simulink model "simulation"  (R2018a)
settings: Solver=VariableStepAuto  StartTime=0.0  StopTime=10.0  RelTol=1e-3
libraries: simulink x6
settings Model: Creator=Migue  LastModifiedBy=Migue
settings SolverCC: AlgebraicLoopSolver=LineSearch

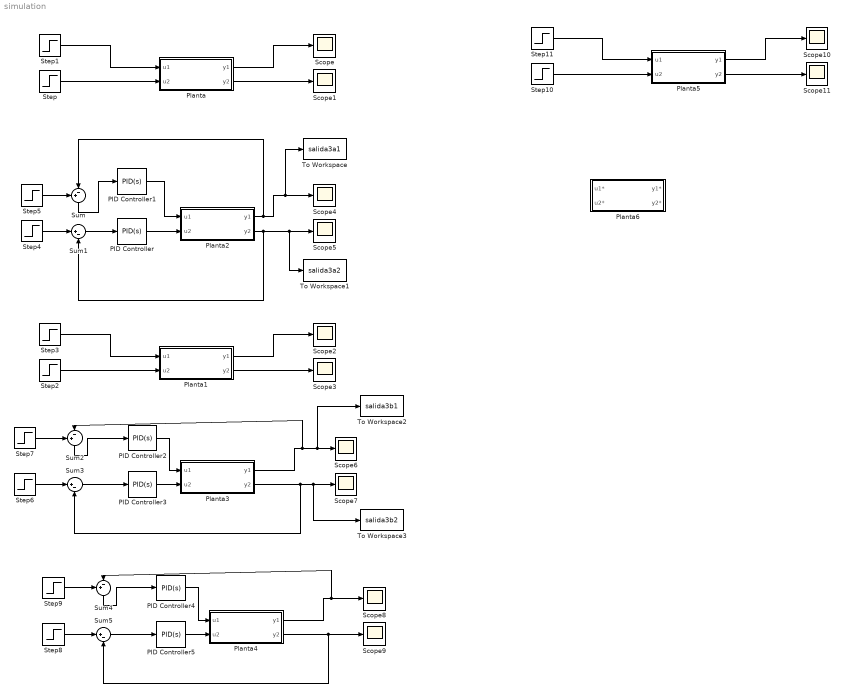
== system simulation ==
  PID Controller : simulink/Continuous/PID Controller  Controller=PID  TimeDomain=Continuous-time  SampleTime=-1  IntegratorMethod=Forward Euler  FilterMethod=Forward Euler  Form=Parallel  UseFilter=on  ControllerParametersSource=internal  P=0  I=19.5  D=0  N=100  InitialConditionSource=internal  InitialConditionForIntegrator=0  InitialConditionForFilter=0  ExternalReset=none  LimitOutput=off  UpperSaturationLimit=inf  LowerSaturationLimit=-inf  LinearizeAsGain=on  AntiWindupMode=none  Kb=1  TrackingMode=off  Kt=1  PParamMin=[]  PParamMax=[]  IParamMin=[]  IParamMax=[]  DParamMin=[]  DParamMax=[]  NParamMin=[]  NParamMax=[]  KbParamMin=[]  KbParamMax=[]  KtParamMin=[]  KtParamMax=[]  POutMin=[]  POutMax=[]  IOutMin=[]  IOutMax=[]  DOutMin=[]  DOutMax=[]  NOutMin=[]  NOutMax=[]  KbOutMin=[]  KbOutMax=[]  KtOutMin=[]  KtOutMax=[]  IntegratorOutMin=[]  IntegratorOutMax=[]  FilterOutMin=[]  FilterOutMax=[]  SumOutMin=[]  SumOutMax=[]  SumI1OutMin=[]  SumI1OutMax=[]  SumI2OutMin=[]  SumI2OutMax=[]  SumI3OutMin=[]  SumI3OutMax=[]  SumDOutMin=[]  SumDOutMax=[]  SaturationOutMin=[]  SaturationOutMax=[]  IntegratorContinuousStateAttributes=''  IntegratorStateMustResolveToSignalObject=off  IntegratorRTWStateStorageClass=Auto  FilterContinuousStateAttributes=''  FilterStateMustResolveToSignalObject=off  FilterRTWStateStorageClass=Auto  DifferentiatorICPrevScaledInput=0  DifferentiatorOutMin=[]  DifferentiatorOutMax=[]  FilterDiffOutCoefMin=[]  FilterDiffOutCoefMax=[]  SumDenOutMin=[]  SumDenOutMax=[]  SumNumOutMin=[]  SumNumOutMax=[]  ReciprocalOutMin=[]  ReciprocalOutMax=[]  DivideOutMin=[]  DivideOutMax=[]  TunerSelectOption=Transfer Function Based (PID Tuner App)
  PID Controller1 : simulink/Continuous/PID Controller  Controller=PID  TimeDomain=Continuous-time  SampleTime=-1  IntegratorMethod=Forward Euler  FilterMethod=Forward Euler  Form=Parallel  UseFilter=on  ControllerParametersSource=internal  P=0  I=9.5  D=0  N=100  InitialConditionSource=internal  InitialConditionForIntegrator=0  InitialConditionForFilter=0  ExternalReset=none  LimitOutput=off  UpperSaturationLimit=inf  LowerSaturationLimit=-inf  LinearizeAsGain=on  AntiWindupMode=none  Kb=1  TrackingMode=off  Kt=1  PParamMin=[]  PParamMax=[]  IParamMin=[]  IParamMax=[]  DParamMin=[]  DParamMax=[]  NParamMin=[]  NParamMax=[]  KbParamMin=[]  KbParamMax=[]  KtParamMin=[]  KtParamMax=[]  POutMin=[]  POutMax=[]  IOutMin=[]  IOutMax=[]  DOutMin=[]  DOutMax=[]  NOutMin=[]  NOutMax=[]  KbOutMin=[]  KbOutMax=[]  KtOutMin=[]  KtOutMax=[]  IntegratorOutMin=[]  IntegratorOutMax=[]  FilterOutMin=[]  FilterOutMax=[]  SumOutMin=[]  SumOutMax=[]  SumI1OutMin=[]  SumI1OutMax=[]  SumI2OutMin=[]  SumI2OutMax=[]  SumI3OutMin=[]  SumI3OutMax=[]  SumDOutMin=[]  SumDOutMax=[]  SaturationOutMin=[]  SaturationOutMax=[]  IntegratorContinuousStateAttributes=''  IntegratorStateMustResolveToSignalObject=off  IntegratorRTWStateStorageClass=Auto  FilterContinuousStateAttributes=''  FilterStateMustResolveToSignalObject=off  FilterRTWStateStorageClass=Auto  DifferentiatorICPrevScaledInput=0  DifferentiatorOutMin=[]  DifferentiatorOutMax=[]  FilterDiffOutCoefMin=[]  FilterDiffOutCoefMax=[]  SumDenOutMin=[]  SumDenOutMax=[]  SumNumOutMin=[]  SumNumOutMax=[]  ReciprocalOutMin=[]  ReciprocalOutMax=[]  DivideOutMin=[]  DivideOutMax=[]  TunerSelectOption=Transfer Function Based (PID Tuner App)
  PID Controller2 : simulink/Continuous/PID Controller  Controller=PID  TimeDomain=Continuous-time  SampleTime=-1  IntegratorMethod=Forward Euler  FilterMethod=Forward Euler  Form=Parallel  UseFilter=on  ControllerParametersSource=internal  P=0.06  I=16.15  D=0  N=100  InitialConditionSource=internal  InitialConditionForIntegrator=0  InitialConditionForFilter=0  ExternalReset=none  LimitOutput=off  UpperSaturationLimit=inf  LowerSaturationLimit=-inf  LinearizeAsGain=on  AntiWindupMode=none  Kb=1  TrackingMode=off  Kt=1  PParamMin=[]  PParamMax=[]  IParamMin=[]  IParamMax=[]  DParamMin=[]  DParamMax=[]  NParamMin=[]  NParamMax=[]  KbParamMin=[]  KbParamMax=[]  KtParamMin=[]  KtParamMax=[]  POutMin=[]  POutMax=[]  IOutMin=[]  IOutMax=[]  DOutMin=[]  DOutMax=[]  NOutMin=[]  NOutMax=[]  KbOutMin=[]  KbOutMax=[]  KtOutMin=[]  KtOutMax=[]  IntegratorOutMin=[]  IntegratorOutMax=[]  FilterOutMin=[]  FilterOutMax=[]  SumOutMin=[]  SumOutMax=[]  SumI1OutMin=[]  SumI1OutMax=[]  SumI2OutMin=[]  SumI2OutMax=[]  SumI3OutMin=[]  SumI3OutMax=[]  SumDOutMin=[]  SumDOutMax=[]  SaturationOutMin=[]  SaturationOutMax=[]  IntegratorContinuousStateAttributes=''  IntegratorStateMustResolveToSignalObject=off  IntegratorRTWStateStorageClass=Auto  FilterContinuousStateAttributes=''  FilterStateMustResolveToSignalObject=off  FilterRTWStateStorageClass=Auto  DifferentiatorICPrevScaledInput=0  DifferentiatorOutMin=[]  DifferentiatorOutMax=[]  FilterDiffOutCoefMin=[]  FilterDiffOutCoefMax=[]  SumDenOutMin=[]  SumDenOutMax=[]  SumNumOutMin=[]  SumNumOutMax=[]  ReciprocalOutMin=[]  ReciprocalOutMax=[]  DivideOutMin=[]  DivideOutMax=[]  TunerSelectOption=Transfer Function Based (PID Tuner App)
  PID Controller3 : simulink/Continuous/PID Controller  Controller=PID  TimeDomain=Continuous-time  SampleTime=-1  IntegratorMethod=Forward Euler  FilterMethod=Forward Euler  Form=Parallel  UseFilter=on  ControllerParametersSource=internal  P=0  I=10  D=0  N=100  InitialConditionSource=internal  InitialConditionForIntegrator=0  InitialConditionForFilter=0  ExternalReset=none  LimitOutput=off  UpperSaturationLimit=inf  LowerSaturationLimit=-inf  LinearizeAsGain=on  AntiWindupMode=none  Kb=1  TrackingMode=off  Kt=1  PParamMin=[]  PParamMax=[]  IParamMin=[]  IParamMax=[]  DParamMin=[]  DParamMax=[]  NParamMin=[]  NParamMax=[]  KbParamMin=[]  KbParamMax=[]  KtParamMin=[]  KtParamMax=[]  POutMin=[]  POutMax=[]  IOutMin=[]  IOutMax=[]  DOutMin=[]  DOutMax=[]  NOutMin=[]  NOutMax=[]  KbOutMin=[]  KbOutMax=[]  KtOutMin=[]  KtOutMax=[]  IntegratorOutMin=[]  IntegratorOutMax=[]  FilterOutMin=[]  FilterOutMax=[]  SumOutMin=[]  SumOutMax=[]  SumI1OutMin=[]  SumI1OutMax=[]  SumI2OutMin=[]  SumI2OutMax=[]  SumI3OutMin=[]  SumI3OutMax=[]  SumDOutMin=[]  SumDOutMax=[]  SaturationOutMin=[]  SaturationOutMax=[]  IntegratorContinuousStateAttributes=''  IntegratorStateMustResolveToSignalObject=off  IntegratorRTWStateStorageClass=Auto  FilterContinuousStateAttributes=''  FilterStateMustResolveToSignalObject=off  FilterRTWStateStorageClass=Auto  DifferentiatorICPrevScaledInput=0  DifferentiatorOutMin=[]  DifferentiatorOutMax=[]  FilterDiffOutCoefMin=[]  FilterDiffOutCoefMax=[]  SumDenOutMin=[]  SumDenOutMax=[]  SumNumOutMin=[]  SumNumOutMax=[]  ReciprocalOutMin=[]  ReciprocalOutMax=[]  DivideOutMin=[]  DivideOutMax=[]  TunerSelectOption=Transfer Function Based (PID Tuner App)
  PID Controller4 : simulink/Continuous/PID Controller  Controller=PID  TimeDomain=Continuous-time  SampleTime=-1  IntegratorMethod=Forward Euler  FilterMethod=Forward Euler  Form=Parallel  UseFilter=on  ControllerParametersSource=internal  P=0.06  I=16.15  D=0  N=100  InitialConditionSource=internal  InitialConditionForIntegrator=0  InitialConditionForFilter=0  ExternalReset=none  LimitOutput=off  UpperSaturationLimit=inf  LowerSaturationLimit=-inf  LinearizeAsGain=on  AntiWindupMode=none  Kb=1  TrackingMode=off  Kt=1  PParamMin=[]  PParamMax=[]  IParamMin=[]  IParamMax=[]  DParamMin=[]  DParamMax=[]  NParamMin=[]  NParamMax=[]  KbParamMin=[]  KbParamMax=[]  KtParamMin=[]  KtParamMax=[]  POutMin=[]  POutMax=[]  IOutMin=[]  IOutMax=[]  DOutMin=[]  DOutMax=[]  NOutMin=[]  NOutMax=[]  KbOutMin=[]  KbOutMax=[]  KtOutMin=[]  KtOutMax=[]  IntegratorOutMin=[]  IntegratorOutMax=[]  FilterOutMin=[]  FilterOutMax=[]  SumOutMin=[]  SumOutMax=[]  SumI1OutMin=[]  SumI1OutMax=[]  SumI2OutMin=[]  SumI2OutMax=[]  SumI3OutMin=[]  SumI3OutMax=[]  SumDOutMin=[]  SumDOutMax=[]  SaturationOutMin=[]  SaturationOutMax=[]  IntegratorContinuousStateAttributes=''  IntegratorStateMustResolveToSignalObject=off  IntegratorRTWStateStorageClass=Auto  FilterContinuousStateAttributes=''  FilterStateMustResolveToSignalObject=off  FilterRTWStateStorageClass=Auto  DifferentiatorICPrevScaledInput=0  DifferentiatorOutMin=[]  DifferentiatorOutMax=[]  FilterDiffOutCoefMin=[]  FilterDiffOutCoefMax=[]  SumDenOutMin=[]  SumDenOutMax=[]  SumNumOutMin=[]  SumNumOutMax=[]  ReciprocalOutMin=[]  ReciprocalOutMax=[]  DivideOutMin=[]  DivideOutMax=[]  TunerSelectOption=Transfer Function Based (PID Tuner App)
  PID Controller5 : simulink/Continuous/PID Controller  Controller=PID  TimeDomain=Continuous-time  SampleTime=-1  IntegratorMethod=Forward Euler  FilterMethod=Forward Euler  Form=Parallel  UseFilter=on  ControllerParametersSource=internal  P=0  I=10  D=0  N=100  InitialConditionSource=internal  InitialConditionForIntegrator=0  InitialConditionForFilter=0  ExternalReset=none  LimitOutput=off  UpperSaturationLimit=inf  LowerSaturationLimit=-inf  LinearizeAsGain=on  AntiWindupMode=none  Kb=1  TrackingMode=off  Kt=1  PParamMin=[]  PParamMax=[]  IParamMin=[]  IParamMax=[]  DParamMin=[]  DParamMax=[]  NParamMin=[]  NParamMax=[]  KbParamMin=[]  KbParamMax=[]  KtParamMin=[]  KtParamMax=[]  POutMin=[]  POutMax=[]  IOutMin=[]  IOutMax=[]  DOutMin=[]  DOutMax=[]  NOutMin=[]  NOutMax=[]  KbOutMin=[]  KbOutMax=[]  KtOutMin=[]  KtOutMax=[]  IntegratorOutMin=[]  IntegratorOutMax=[]  FilterOutMin=[]  FilterOutMax=[]  SumOutMin=[]  SumOutMax=[]  SumI1OutMin=[]  SumI1OutMax=[]  SumI2OutMin=[]  SumI2OutMax=[]  SumI3OutMin=[]  SumI3OutMax=[]  SumDOutMin=[]  SumDOutMax=[]  SaturationOutMin=[]  SaturationOutMax=[]  IntegratorContinuousStateAttributes=''  IntegratorStateMustResolveToSignalObject=off  IntegratorRTWStateStorageClass=Auto  FilterContinuousStateAttributes=''  FilterStateMustResolveToSignalObject=off  FilterRTWStateStorageClass=Auto  DifferentiatorICPrevScaledInput=0  DifferentiatorOutMin=[]  DifferentiatorOutMax=[]  FilterDiffOutCoefMin=[]  FilterDiffOutCoefMax=[]  SumDenOutMin=[]  SumDenOutMax=[]  SumNumOutMin=[]  SumNumOutMax=[]  ReciprocalOutMin=[]  ReciprocalOutMax=[]  DivideOutMin=[]  DivideOutMax=[]  TunerSelectOption=Transfer Function Based (PID Tuner App)
  Planta : Subsystem
  Planta1 : Subsystem
  Planta2 : Subsystem
  Planta3 : Subsystem
  Planta4 : Subsystem
  Planta5 : Subsystem
  Planta6 : Subsystem
  Scope{,1..11} (12 alike) : Scope
  Step{,1..11} (12 alike) : Step  SampleTime=0
  Sum : Sum  Inputs=+-|
  Sum1 : Sum  Inputs=|+-
  Sum2 : Sum  Inputs=+-|
  Sum3 : Sum  Inputs=|+-
  Sum4 : Sum  Inputs=+-|
  Sum5 : Sum  Inputs=|+-
  To Workspace : ToWorkspace  VariableName=salida3a1  SaveFormat=Timeseries  SampleTime=-1
  To Workspace1 : ToWorkspace  VariableName=salida3a2  SaveFormat=Timeseries  SampleTime=-1
  To Workspace2 : ToWorkspace  VariableName=salida3b1  SaveFormat=Timeseries  SampleTime=-1
  To Workspace3 : ToWorkspace  VariableName=salida3b2  SaveFormat=Timeseries  SampleTime=-1
  wires:
  Step1/1 -> Planta/1(u1)
  Step/1 -> Planta/2(u2)
  Planta/2(y2) -> Scope1/1
  Planta/1(y1) -> Scope/1
  Planta1/1(y1) -> Scope2/1
  Step2/1 -> Planta1/2(u2)
  Step3/1 -> Planta1/1(u1)
  Planta1/2(y2) -> Scope3/1
  Planta2/1(y1) -> Sum/2, To Workspace/1, Scope4/1
  Planta2/2(y2) -> Sum1/2, To Workspace1/1, Scope5/1
  Step5/1 -> Sum/1
  Step4/1 -> Sum1/1
  Sum1/1 -> PID Controller/1
  PID Controller/1 -> Planta2/2(u2)
  PID Controller1/1 -> Planta2/1(u1)
  Sum/1 -> PID Controller1/1
  Planta3/2(y2) -> Sum3/2, To Workspace3/1, Scope7/1
  Planta3/1(y1) -> Sum2/2, To Workspace2/1, Scope6/1
  PID Controller3/1 -> Planta3/2(u2)
  PID Controller2/1 -> Planta3/1(u1)
  Sum3/1 -> PID Controller3/1
  Step6/1 -> Sum3/1
  Sum2/1 -> PID Controller2/1
  Step7/1 -> Sum2/1
  Step8/1 -> Sum5/1
  PID Controller5/1 -> Planta4/2(u2)
  Sum4/1 -> PID Controller4/1
  Step9/1 -> Sum4/1
  Planta4/2(y2) -> Sum5/2, Scope9/1
  Sum5/1 -> PID Controller5/1
  Planta4/1(y1) -> Sum4/2, Scope8/1
  PID Controller4/1 -> Planta4/1(u1)
  Planta5/1(y1) -> Scope10/1
  Step10/1 -> Planta5/2(u2)
  Step11/1 -> Planta5/1(u1)
  Planta5/2(y2) -> Scope11/1

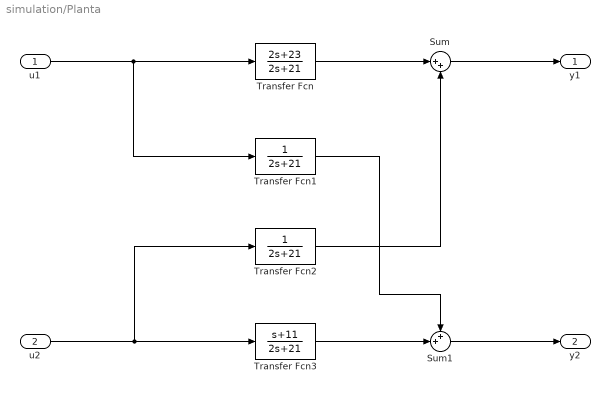
== system simulation/Planta ==
  u1 : Inport
  u2 : Inport  Port=2
  Sum : Sum  Inputs=|++
  Sum1 : Sum  Inputs=++|
  Transfer Fcn : TransferFcn  Numerator=[2 23]  Denominator=[2 21]
  Transfer Fcn1 : TransferFcn  Denominator=[2 21]
  Transfer Fcn2 : TransferFcn  Denominator=[2 21]
  Transfer Fcn3 : TransferFcn  Numerator=[1 11]  Denominator=[2 21]
  y1 : Outport
  y2 : Outport  Port=2
  wires:
  u1/1 -> Transfer Fcn1/1, Transfer Fcn/1
  u2/1 -> Transfer Fcn2/1, Transfer Fcn3/1
  Transfer Fcn3/1 -> Sum1/2
  Transfer Fcn/1 -> Sum/1
  Transfer Fcn2/1 -> Sum/2
  Transfer Fcn1/1 -> Sum1/1
  Sum1/1 -> y2/1
  Sum/1 -> y1/1

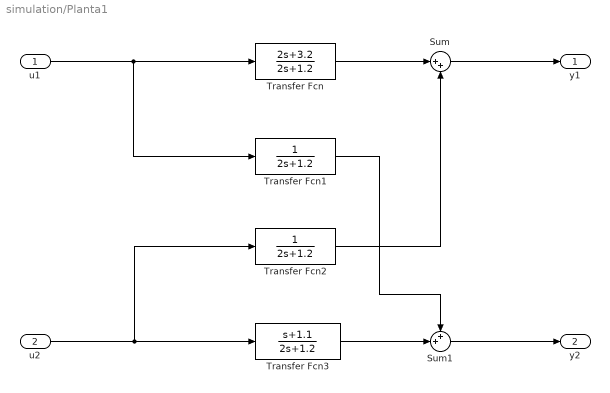
== system simulation/Planta1 ==
  u1 : Inport
  u2 : Inport  Port=2
  Sum : Sum  Inputs=|++
  Sum1 : Sum  Inputs=++|
  Transfer Fcn : TransferFcn  Numerator=[2 3.2]  Denominator=[2 1.2]
  Transfer Fcn1 : TransferFcn  Denominator=[2 1.2]
  Transfer Fcn2 : TransferFcn  Denominator=[2 1.2]
  Transfer Fcn3 : TransferFcn  Numerator=[1 1.1]  Denominator=[2 1.2]
  y1 : Outport
  y2 : Outport  Port=2
  wires:
  u1/1 -> Transfer Fcn1/1, Transfer Fcn/1
  u2/1 -> Transfer Fcn2/1, Transfer Fcn3/1
  Transfer Fcn3/1 -> Sum1/2
  Transfer Fcn/1 -> Sum/1
  Transfer Fcn2/1 -> Sum/2
  Transfer Fcn1/1 -> Sum1/1
  Sum1/1 -> y2/1
  Sum/1 -> y1/1

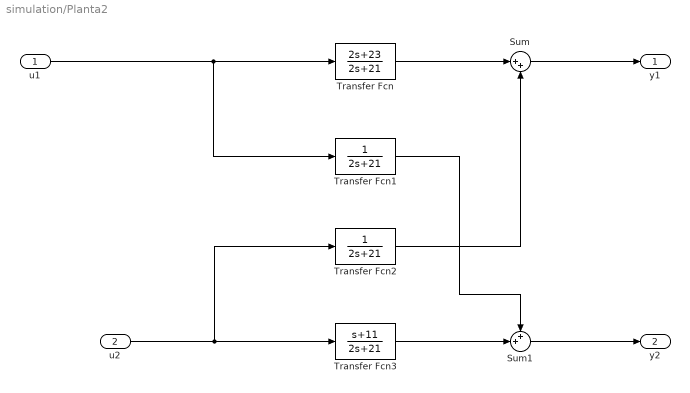
== system simulation/Planta2 ==
  u1 : Inport
  u2 : Inport  Port=2
  Sum : Sum  Inputs=|++
  Sum1 : Sum  Inputs=++|
  Transfer Fcn : TransferFcn  Numerator=[2 23]  Denominator=[2 21]
  Transfer Fcn1 : TransferFcn  Denominator=[2 21]
  Transfer Fcn2 : TransferFcn  Denominator=[2 21]
  Transfer Fcn3 : TransferFcn  Numerator=[1 11]  Denominator=[2 21]
  y1 : Outport
  y2 : Outport  Port=2
  wires:
  u1/1 -> Transfer Fcn1/1, Transfer Fcn/1
  u2/1 -> Transfer Fcn2/1, Transfer Fcn3/1
  Transfer Fcn3/1 -> Sum1/2
  Transfer Fcn/1 -> Sum/1
  Transfer Fcn2/1 -> Sum/2
  Transfer Fcn1/1 -> Sum1/1
  Sum1/1 -> y2/1
  Sum/1 -> y1/1

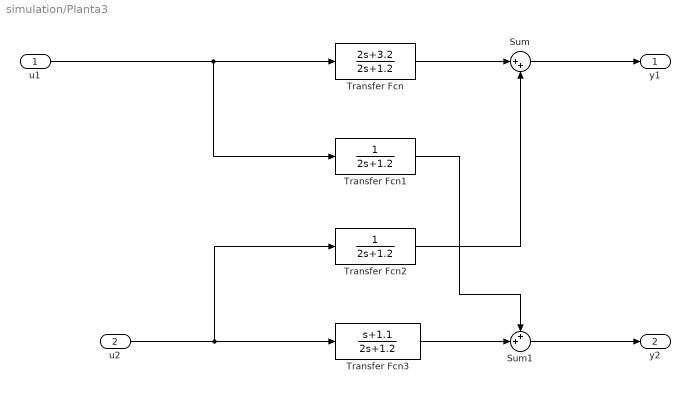
== system simulation/Planta3 ==
  u1 : Inport
  u2 : Inport  Port=2
  Sum : Sum  Inputs=|++
  Sum1 : Sum  Inputs=++|
  Transfer Fcn : TransferFcn  Numerator=[2 3.2]  Denominator=[2 1.2]
  Transfer Fcn1 : TransferFcn  Denominator=[2 1.2]
  Transfer Fcn2 : TransferFcn  Denominator=[2 1.2]
  Transfer Fcn3 : TransferFcn  Numerator=[1 1.1]  Denominator=[2 1.2]
  y1 : Outport
  y2 : Outport  Port=2
  wires:
  u1/1 -> Transfer Fcn1/1, Transfer Fcn/1
  u2/1 -> Transfer Fcn2/1, Transfer Fcn3/1
  Transfer Fcn3/1 -> Sum1/2
  Transfer Fcn/1 -> Sum/1
  Transfer Fcn2/1 -> Sum/2
  Transfer Fcn1/1 -> Sum1/1
  Sum1/1 -> y2/1
  Sum/1 -> y1/1

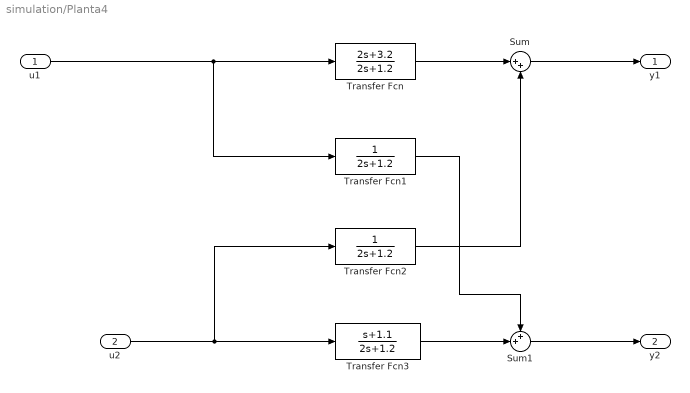
== system simulation/Planta4 ==
  u1 : Inport
  u2 : Inport  Port=2
  Sum : Sum  Inputs=|++
  Sum1 : Sum  Inputs=++|
  Transfer Fcn : TransferFcn  Numerator=[2 3.2]  Denominator=[2 1.2]
  Transfer Fcn1 : TransferFcn  Denominator=[2 1.2]
  Transfer Fcn2 : TransferFcn  Denominator=[2 1.2]
  Transfer Fcn3 : TransferFcn  Numerator=[1 1.1]  Denominator=[2 1.2]
  y1 : Outport
  y2 : Outport  Port=2
  wires:
  u1/1 -> Transfer Fcn1/1, Transfer Fcn/1
  u2/1 -> Transfer Fcn2/1, Transfer Fcn3/1
  Transfer Fcn3/1 -> Sum1/2
  Transfer Fcn/1 -> Sum/1
  Transfer Fcn2/1 -> Sum/2
  Transfer Fcn1/1 -> Sum1/1
  Sum1/1 -> y2/1
  Sum/1 -> y1/1

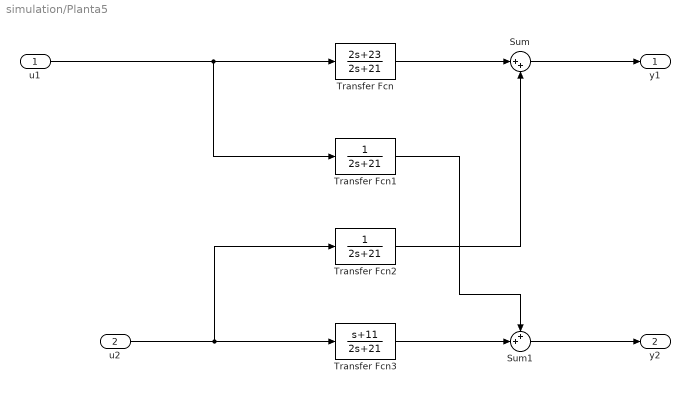
== system simulation/Planta5 ==
  u1 : Inport
  u2 : Inport  Port=2
  Sum : Sum  Inputs=|++
  Sum1 : Sum  Inputs=++|
  Transfer Fcn : TransferFcn  Numerator=[2 23]  Denominator=[2 21]
  Transfer Fcn1 : TransferFcn  Denominator=[2 21]
  Transfer Fcn2 : TransferFcn  Denominator=[2 21]
  Transfer Fcn3 : TransferFcn  Numerator=[1 11]  Denominator=[2 21]
  y1 : Outport
  y2 : Outport  Port=2
  wires:
  u1/1 -> Transfer Fcn1/1, Transfer Fcn/1
  u2/1 -> Transfer Fcn2/1, Transfer Fcn3/1
  Transfer Fcn3/1 -> Sum1/2
  Transfer Fcn/1 -> Sum/1
  Transfer Fcn2/1 -> Sum/2
  Transfer Fcn1/1 -> Sum1/1
  Sum1/1 -> y2/1
  Sum/1 -> y1/1

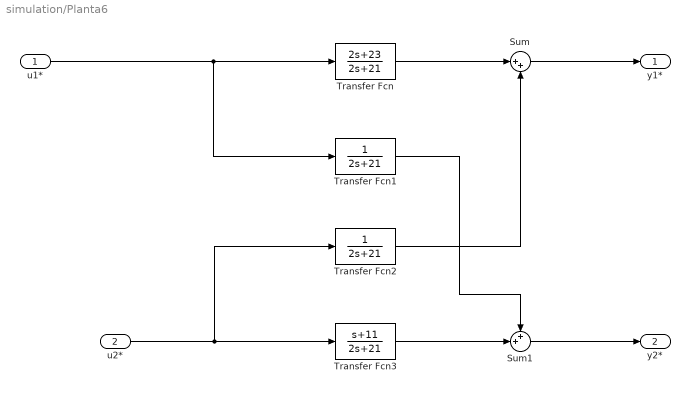
== system simulation/Planta6 ==
  u1* : Inport
  "u2* " : Inport  Port=2
  Sum : Sum  Inputs=|++
  Sum1 : Sum  Inputs=++|
  Transfer Fcn : TransferFcn  Numerator=[2 23]  Denominator=[2 21]
  Transfer Fcn1 : TransferFcn  Denominator=[2 21]
  Transfer Fcn2 : TransferFcn  Denominator=[2 21]
  Transfer Fcn3 : TransferFcn  Numerator=[1 11]  Denominator=[2 21]
  "y1* " : Outport
  y2* : Outport  Port=2
  wires:
  u1*/1 -> Transfer Fcn1/1, Transfer Fcn/1
  "u2* "/1 -> Transfer Fcn2/1, Transfer Fcn3/1
  Transfer Fcn3/1 -> Sum1/2
  Transfer Fcn/1 -> Sum/1
  Transfer Fcn2/1 -> Sum/2
  Transfer Fcn1/1 -> Sum1/1
  Sum1/1 -> y2*/1
  Sum/1 -> "y1* "/1
